simulink model "UnTrans_nonLmodel"  (R2015a)
settings: Solver=ode3  StartTime=0.0  StopTime=20.0  FixedStep=0.01  MaxStep=0.001  RelTol=1e-3
values from neighbouring files (symbols this model uses):
  K2 = K2/10    [try_checkstuff_BUN.m]
undefined symbols (not defined in the file or in its folder): NL
settings Model: CovSFcnEnable=off  Creator=Dawid  LastModifiedBy=Maria
settings DataIOCC: SignalLoggingSaveFormat=ModelDataLogs
settings OptimizationCC: ExpressionDepthLimit=2147483647
settings DebuggingCC: UnderspecifiedInitializationDetection=Classic  MergeDetectMultiDrivingBlocksExec=none  SolverPrmCheckMsg=warning  FcnCallInpInsideContextMsg=UseLocalSettings  StateNameClashWarn=warning
settings GRTTargetCC: CombineOutputUpdateFcns=off  GRTInterface=on

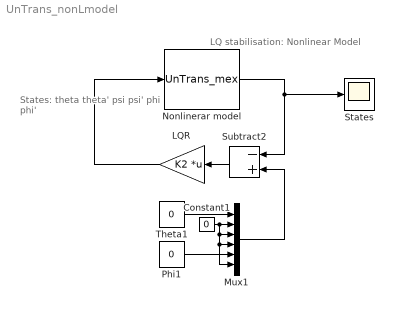
== system UnTrans_nonLmodel ==
  note: States:
      | theta
      | theta'
      | psi
      | psi'
      | phi
      | phi'
  note: LQ stabilisation: Nonlinear Model
  Constant1 : Constant  Value=0
  LQR : Gain  Gain=K2  Multiplication=Matrix(K*u)
  Mux1 : Mux  Inputs=6
  Nonlinerar model : S-Function  InitFcn=|  FunctionName=UnTrans_mex  Parameters=x0, [NL.d1, NL.d2, NL.c1, NL.c2, NL.c3, NL.Jd, NL.MRL, NL.MLL, NL.MgL, NL.W2R, NL.Ffw]  mask(S-function: untrans){x0=[0 0 0.1 0 0 0], NL=NL}
      | UnTransPar = UnTransParams( );           
      | [NL] = UnTransNonlinearModel(UnTransPar);
      mask prompts: x0 "Initial conditions: [theta, theta',psi,psi',phi,phi']"; NL "Model Parameters"
      mask help:
      | This is a S-function block which implements
      | nonlinear model of two wheeled balancing robot.
      mask Display: image( imread('Trans_non.jpg','jpg') )
  Phi1 : Constant  Value=0
  States : Scope
      settings: YMax=12  SaveName=Data_sim_nl
  Subtract2 : Sum  Inputs=-+
  Theta1 : Constant  Value=0
  wires:
  Nonlinerar model/1 -> Subtract2/1, States/1
  LQR/1 -> Nonlinerar model/1
  Theta1/1 -> Mux1/1
  Phi1/1 -> Mux1/5
  Constant1/1 -> Mux1/6, Mux1/4, Mux1/3, Mux1/2
  Subtract2/1 -> LQR/1
  Mux1/1 -> Subtract2/2
